simulink model "rover_cold"  (R2021a)
settings: Solver=VariableStepAuto  StartTime=0.0  StopTime=43200  RelTol=1e-3
libraries: fl_lib x22, nesl_utility x4
settings Model: Creator=dinen  LastModifiedBy=dinen

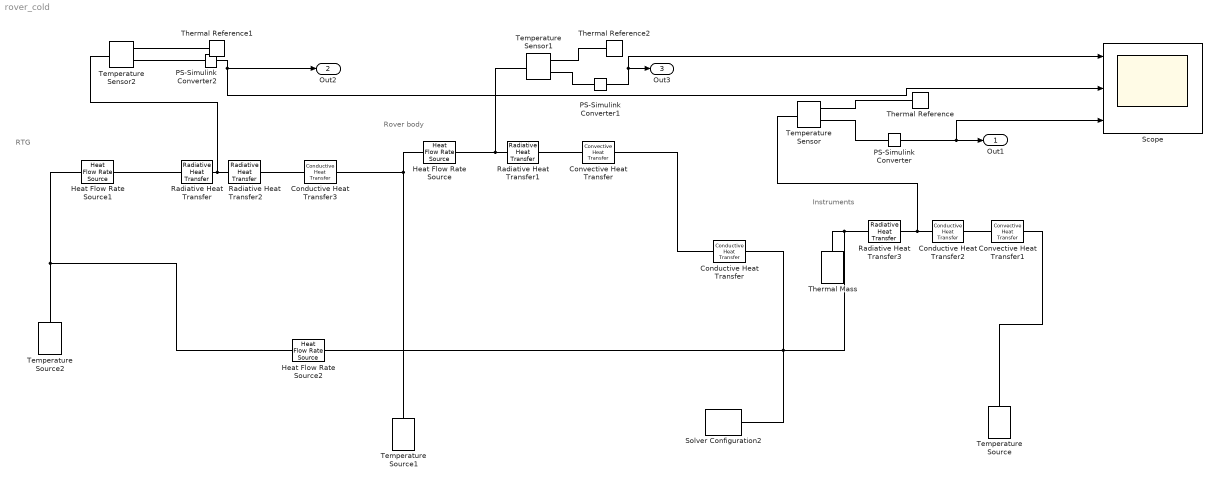
== system rover_cold ==
  note: Instruments
  note: RTG
  note: Rover body
  Conductive Heat Transfer : fl_lib/Thermal/Thermal Elements/Conductive Heat Transfer  area=2.2435 m^2  thickness=0.7 m  th_cond=130 W/(m*K)  T_specify=off  T_priority=None  T=0 K  T_nominal_specify=off  T_nominal_unit=K  T_nominal_value=1  Q_specify=off  Q_priority=None  Q=0 W  Q_nominal_specify=off  Q_nominal_unit=W  Q_nominal_value=1
  Conductive Heat Transfer2 : fl_lib/Thermal/Thermal Elements/Conductive Heat Transfer  area=2.1 m^2  thickness=0.7 m  th_cond=120 W/(m*K)  T_specify=off  T_priority=None  T=0 K  T_nominal_specify=off  T_nominal_unit=K  T_nominal_value=1  Q_specify=off  Q_priority=None  Q=0 W  Q_nominal_specify=off  Q_nominal_unit=W  Q_nominal_value=1
  Conductive Heat Transfer3 : fl_lib/Thermal/Thermal Elements/Conductive Heat Transfer  area=1.074 m^2  thickness=0.016 m  th_cond=0.015 W/(m*K)  T_specify=off  T_priority=None  T=0 K  T_nominal_specify=off  T_nominal_unit=K  T_nominal_value=1  Q_specify=off  Q_priority=None  Q=0 W  Q_nominal_specify=off  Q_nominal_unit=W  Q_nominal_value=1
  Convective Heat Transfer : fl_lib/Thermal/Thermal Elements/Convective Heat Transfer  area=2.2435 m^2  heat_tr_coeff=1 W/(m^2 * K)  T_specify=off  T_priority=None  T=0 K  T_nominal_specify=off  T_nominal_unit=K  T_nominal_value=1  Q_specify=off  Q_priority=None  Q=0 W  Q_nominal_specify=off  Q_nominal_unit=W  Q_nominal_value=1
  Convective Heat Transfer1 : fl_lib/Thermal/Thermal Elements/Convective Heat Transfer  area=2.1 m^2  heat_tr_coeff=1 W/(m^2 * K)  T_specify=off  T_priority=None  T=0 K  T_nominal_specify=off  T_nominal_unit=K  T_nominal_value=1  Q_specify=off  Q_priority=None  Q=0 W  Q_nominal_specify=off  Q_nominal_unit=W  Q_nominal_value=1
  Heat Flow Rate Source : fl_lib/Thermal/Thermal Sources/Heat Flow Rate Source  heat_flow=33.4 W
      settings: SourceProductBaseCode=SS  InternalSimscapePortConfiguration="{\"Bottom\":[],\"Left\":[{\"id\":\"B\",\"label\":\"B\",\"type\":\"foundation.thermal.thermal\"}],\"Right\":[{\"id\":\"A\",\"label\":\"A\",\"type\":\"foundation.thermal.thermal\"}],\"Top\":[]}"
  Heat Flow Rate Source1 : fl_lib/Thermal/Thermal Sources/Heat Flow Rate Source  heat_flow=145 W
      settings: SourceProductBaseCode=SS  InternalSimscapePortConfiguration="{\"Bottom\":[],\"Left\":[{\"id\":\"B\",\"label\":\"B\",\"type\":\"foundation.thermal.thermal\"}],\"Right\":[{\"id\":\"A\",\"label\":\"A\",\"type\":\"foundation.thermal.thermal\"}],\"Top\":[]}"
  Heat Flow Rate Source2 : fl_lib/Thermal/Thermal Sources/Heat Flow Rate Source  heat_flow=30 W
      settings: SourceProductBaseCode=SS  InternalSimscapePortConfiguration="{\"Bottom\":[],\"Left\":[{\"id\":\"B\",\"label\":\"B\",\"type\":\"foundation.thermal.thermal\"}],\"Right\":[{\"id\":\"A\",\"label\":\"A\",\"type\":\"foundation.thermal.thermal\"}],\"Top\":[]}"
  PS-Simulink Converter : nesl_utility/PS-Simulink Converter  PhysicalDomain=network_engine_domain  SubClassName=ps_output  LeftPortType=input  RightPortType=output  PseudoPeriodic=off  Frequencies=[]  Unit=inherit  AffineConversion=off
      settings: SourceProductBaseCode=PW,SS
  PS-Simulink Converter1 : nesl_utility/PS-Simulink Converter  PhysicalDomain=network_engine_domain  SubClassName=ps_output  LeftPortType=input  RightPortType=output  PseudoPeriodic=off  Frequencies=[]  Unit=inherit  AffineConversion=off
      settings: SourceProductBaseCode=PW,SS
  PS-Simulink Converter2 : nesl_utility/PS-Simulink Converter  PhysicalDomain=network_engine_domain  SubClassName=ps_output  LeftPortType=input  RightPortType=output  PseudoPeriodic=off  Frequencies=[]  Unit=inherit  AffineConversion=off
      settings: SourceProductBaseCode=PW,SS
  Radiative Heat Transfer : fl_lib/Thermal/Thermal Elements/Radiative Heat Transfer  area=1.6525 m^2  rad_tr_coeff=0.9245 W/(m^2*K^4)  T_specify=off  T_priority=None  T=0 K  T_nominal_specify=off  T_nominal_unit=K  T_nominal_value=1  Q_specify=off  Q_priority=None  Q=0 W  Q_nominal_specify=off  Q_nominal_unit=W  Q_nominal_value=1
      settings: SourceProductBaseCode=SS  InternalSimscapePortConfiguration="{\"Bottom\":[],\"Left\":[{\"id\":\"A\",\"label\":\"A\",\"type\":\"foundation.thermal.thermal\"}],\"Right\":[{\"id\":\"B\",\"label\":\"B\",\"type\":\"foundation.thermal.thermal\"}],\"Top\":[]}"
  Radiative Heat Transfer1 : fl_lib/Thermal/Thermal Elements/Radiative Heat Transfer  area=2.2435 m^2  rad_tr_coeff=1.25636 W/(m^2*K^4)  T_specify=off  T_priority=None  T=0 K  T_nominal_specify=off  T_nominal_unit=K  T_nominal_value=1  Q_specify=off  Q_priority=None  Q=0 W  Q_nominal_specify=off  Q_nominal_unit=W  Q_nominal_value=1
      settings: SourceProductBaseCode=SS  InternalSimscapePortConfiguration="{\"Bottom\":[],\"Left\":[{\"id\":\"A\",\"label\":\"A\",\"type\":\"foundation.thermal.thermal\"}],\"Right\":[{\"id\":\"B\",\"label\":\"B\",\"type\":\"foundation.thermal.thermal\"}],\"Top\":[]}"
  Radiative Heat Transfer2 : fl_lib/Thermal/Thermal Elements/Radiative Heat Transfer  area=1.074 m^2  rad_tr_coeff=0.0113 W/(m^2*K^4)  T_specify=off  T_priority=None  T=0 K  T_nominal_specify=off  T_nominal_unit=K  T_nominal_value=1  Q_specify=off  Q_priority=None  Q=0 W  Q_nominal_specify=off  Q_nominal_unit=W  Q_nominal_value=1
      settings: SourceProductBaseCode=SS  InternalSimscapePortConfiguration="{\"Bottom\":[],\"Left\":[{\"id\":\"A\",\"label\":\"A\",\"type\":\"foundation.thermal.thermal\"}],\"Right\":[{\"id\":\"B\",\"label\":\"B\",\"type\":\"foundation.thermal.thermal\"}],\"Top\":[]}"
  Radiative Heat Transfer3 : fl_lib/Thermal/Thermal Elements/Radiative Heat Transfer  area=2.1 m^2  rad_tr_coeff=1.176 W/(m^2*K^4)  T_specify=off  T_priority=None  T=0 K  T_nominal_specify=off  T_nominal_unit=K  T_nominal_value=1  Q_specify=off  Q_priority=None  Q=0 W  Q_nominal_specify=off  Q_nominal_unit=W  Q_nominal_value=1
      settings: SourceProductBaseCode=SS  InternalSimscapePortConfiguration="{\"Bottom\":[],\"Left\":[{\"id\":\"A\",\"label\":\"A\",\"type\":\"foundation.thermal.thermal\"}],\"Right\":[{\"id\":\"B\",\"label\":\"B\",\"type\":\"foundation.thermal.thermal\"}],\"Top\":[]}"
  Scope : Scope  NumInputPorts=3
  Solver Configuration2 : nesl_utility/Solver Configuration  PhysicalDomain=network_engine_domain  SubClassName=solver  LeftPortType=input  RightPortType=generic  Tones=[]  Harmonics=[]  SimulateNoise=off  Profile=off  UseLocalSampling=off  EnableSwitchedLinearOptims=on  FrequencyDomain=off  UseCCode=off  RelTol=0.001  AbsTol=1e-06  MinStep=1e-09  ToWorkspace=off  RevertToSquareIcSolve=off  NumHomotopyIterations=100  PhasorMode=off  PhasorModeNumHarmonics=1  DoDC=off  ResidualTolerance=1e-09  UseLocalSolver=off  LocalSolverChoice=NE_BACKWARD_EULER_ADVANCER  LocalSolverSampleTime=0.001  DoFixedCost=off  MaxNonlinIter=3  MaxModeIter=2  ComputeImpulses=off  ImpulseIterations=2  LinearAlgebra=auto  EquationFormulation=NE_TIME_EF  DelaysMemoryBudget=1024  AutomaticFiltering=on  FilteringTimeConstant=0.001  PartitionStorageMethod=AS_NEEDED  PartitionMemoryBudget=1024  PartitionMethod=ROBUST
      settings: SourceProductBaseCode=PW,SS
  Temperature Sensor : fl_lib/Thermal/Thermal Sensors/Temperature Sensor
  Temperature Sensor1 : fl_lib/Thermal/Thermal Sensors/Temperature Sensor
  Temperature Sensor2 : fl_lib/Thermal/Thermal Sensors/Temperature Sensor
  Temperature Source : fl_lib/Thermal/Thermal Sources/Temperature Source  temperature=243 K
  Temperature Source1 : fl_lib/Thermal/Thermal Sources/Temperature Source  temperature=243 K
  Temperature Source2 : fl_lib/Thermal/Thermal Sources/Temperature Source  temperature=243 K
  Thermal Mass : fl_lib/Thermal/Thermal Elements/Thermal Mass  mass=26.3 kg  sp_heat=903 J/kg/K  T_specify=on  T_priority=High  T=300 K  T_nominal_specify=off  T_nominal_unit=K  T_nominal_value=1  Q_specify=on  Q_priority=Low  Q=0 W  Q_nominal_specify=off  Q_nominal_unit=W  Q_nominal_value=1
  Thermal Reference : fl_lib/Thermal/Thermal Elements/Thermal Reference
  Thermal Reference1 : fl_lib/Thermal/Thermal Elements/Thermal Reference
  Thermal Reference2 : fl_lib/Thermal/Thermal Elements/Thermal Reference
  Out1 : Outport
  Out2 : Outport  Port=2
  Out3 : Outport  Port=3
  wires:
  PS-Simulink Converter/1 -> Scope/3, Out1/1
  PS-Simulink Converter2/1 -> Out2/1, Scope/2
  PS-Simulink Converter1/1 -> Scope/1, Out3/1
  connections:
  Heat Flow Rate Source1/LConn1 -- Radiative Heat Transfer/LConn1
  Convective Heat Transfer/RConn1 -- Conductive Heat Transfer/LConn1
  Convective Heat Transfer1/RConn1 -- Temperature Source/LConn1
  Temperature Sensor/RConn1 -- Thermal Reference/LConn1
  Temperature Sensor/RConn2 -- PS-Simulink Converter/LConn1
  Radiative Heat Transfer1/RConn1 -- Convective Heat Transfer/LConn1
  Heat Flow Rate Source/RConn1 -- Conductive Heat Transfer3/RConn1 -- Temperature Source1/LConn1
  Radiative Heat Transfer3/LConn1 -- Conductive Heat Transfer/RConn1 -- Heat Flow Rate Source2/LConn1 -- Solver Configuration2/RConn1 -- Thermal Mass/LConn1
  Conductive Heat Transfer2/LConn1 -- Temperature Sensor/LConn1 -- Radiative Heat Transfer3/RConn1
  Convective Heat Transfer1/LConn1 -- Conductive Heat Transfer2/RConn1
  Heat Flow Rate Source/LConn1 -- Temperature Sensor1/LConn1 -- Radiative Heat Transfer1/LConn1
  Heat Flow Rate Source1/RConn1 -- Heat Flow Rate Source2/RConn1 -- Temperature Source2/LConn1
  Radiative Heat Transfer/RConn1 -- Temperature Sensor2/LConn1 -- Radiative Heat Transfer2/LConn1
  Conductive Heat Transfer3/LConn1 -- Radiative Heat Transfer2/RConn1
  Temperature Sensor2/RConn1 -- Thermal Reference1/LConn1
  Temperature Sensor1/RConn1 -- Thermal Reference2/LConn1
  Temperature Sensor2/RConn2 -- PS-Simulink Converter2/LConn1
  Temperature Sensor1/RConn2 -- PS-Simulink Converter1/LConn1
